simulink model "CrCtl_StM"  (R2016b)
settings: configuration reference "CodeGenConfigSet" (kept outside this file)
values from neighbouring files (symbols this model uses):
  CrCtl_aAccThres_C = Calibration.Parameter    [init_CrCtl_StM.m]
  CrCtl_aDeclThres_C = Calibration.Parameter    [init_CrCtl_StM.m]
  CrCtl_facRmpSlpAcc_C = Calibration.Parameter    [init_CrCtl_StM.m]
  CrCtl_facRmpSlpDecl_C = Calibration.Parameter    [init_CrCtl_StM.m]
  CrCtl_facRmpSlpRes_C = Calibration.Parameter    [init_CrCtl_StM.m]
  CrCtl_swtOffTipDwnTrqLim_C = Calibration.Parameter    [init_CrCtl_StM.m]
  CrCtl_swtOffTipUpTrqLim_C = Calibration.Parameter    [init_CrCtl_StM.m]
  CrCtl_trqLimOffsetAcc_C = Calibration.Parameter    [init_CrCtl_StM.m]
  CrCtl_trqLimOffsetDecl_C = Calibration.Parameter    [init_CrCtl_StM.m]
  CrCtl_vDvtMaxAccDecl_C = Calibration.Parameter    [init_CrCtl_StM.m]
  CrCtl_vMaxDvtAcc_C = Calibration.Parameter    [init_CrCtl_StM.m]
  CrCtl_vMaxDvtDecl_C = Calibration.Parameter    [init_CrCtl_StM.m]
  CrCtl_vMaxDvtResAbv_C = Calibration.Parameter    [init_CrCtl_StM.m]
  CrCtl_vMaxDvtResBlw_C = Calibration.Parameter    [init_CrCtl_StM.m]
  CrCtl_vTipDwnDvtn_C = Calibration.Parameter    [init_CrCtl_StM.m]
  CrCtl_vTipDwnLoLim_C = Calibration.Parameter    [init_CrCtl_StM.m]
  CrCtl_vTipDwnUpLim_C = Calibration.Parameter    [init_CrCtl_StM.m]
  CrCtl_vTipStp_C = Calibration.Parameter    [init_CrCtl_StM.m]
  CrCtl_vTipUpDvtn_C = Calibration.Parameter    [init_CrCtl_StM.m]
  CrCtl_vTipUpLoLim_C = Calibration.Parameter    [init_CrCtl_StM.m]
  CrCtl_vTipUpUpLim_C = Calibration.Parameter    [init_CrCtl_StM.m]
  MoFDrAs_vCCtlMinCalMsg_C = Calibration.Parameter    [init_CrCtl_StM.m]
  VEL_ZERO = fi(0,VehSpeed_km_h)    [init_CrCtl_StM.m]
undefined symbols (not defined in the file or in its folder): CrCtl_stLck_conv, CrCtl_StM_DT, CrCtl_stShOff_conv, CrCtl_stSub_conv, CruiseCtl_State_conv
libraries: CXLib x15
(part 2 of 2)

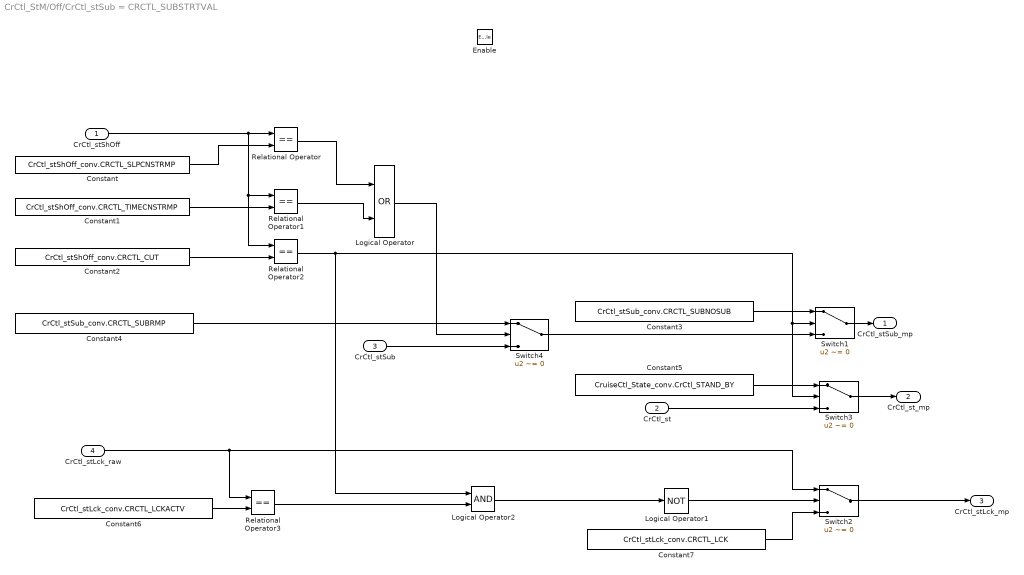
== system CrCtl_StM/Off/CrCtl_stSub = CRCTL_SUBSTRTVAL ==
  "CrCtl_stShOff " : Inport
  CrCtl_st : Inport  Port=2
  CrCtl_stSub : Inport  Port=3
  CrCtl_stLck_raw : Inport  Port=4
  Enable : EnablePort
  Constant : Constant  Value=CrCtl_stShOff_conv.CRCTL_SLPCNSTRMP
  Constant1 : Constant  Value=CrCtl_stShOff_conv.CRCTL_TIMECNSTRMP
  Constant2 : Constant  Value=CrCtl_stShOff_conv.CRCTL_CUT
  Constant3 : Constant  Value=CrCtl_stSub_conv.CRCTL_SUBNOSUB
  Constant4 : Constant  Value=CrCtl_stSub_conv.CRCTL_SUBRMP
  Constant5 : Constant  Value=CruiseCtl_State_conv.CrCtl_STAND_BY
  Constant6 : Constant  Value=CrCtl_stLck_conv.CRCTL_LCKACTV
  Constant7 : Constant  Value=CrCtl_stLck_conv.CRCTL_LCK
  Logical Operator : Logic  Operator=OR  AllPortsSameDT=off  OutDataTypeStr=boolean
  Logical Operator1 : Logic  Operator=NOT  AllPortsSameDT=off  OutDataTypeStr=boolean
  Logical Operator2 : Logic  AllPortsSameDT=off  OutDataTypeStr=boolean
  Relational Operator{,1..3} (4 alike) : RelationalOperator  Operator===  OutDataTypeStr=boolean  RndMeth=Simplest
  Switch{1..4} (4 alike) : Switch  Criteria=u2 ~= 0
  CrCtl_stSub_mp : Outport
  CrCtl_st_mp : Outport  Port=2
  CrCtl_stLck_mp : Outport  Port=3
  wires:
  Relational Operator1/1 -> Logical Operator/2
  Constant4/1 -> Switch4/1
  Switch4/1 -> Switch1/3
  Relational Operator2/1 -> Switch1/2, Switch3/2, Logical Operator2/1
  Constant3/1 -> Switch1/1
  Switch3/1 -> CrCtl_st_mp/1
  Constant7/1 -> Switch2/3
  Logical Operator/1 -> Switch4/2
  Constant5/1 -> Switch3/1
  Switch1/1 -> CrCtl_stSub_mp/1
  CrCtl_stLck_raw/1 -> Relational Operator3/1, Switch2/1
  Relational Operator/1 -> Logical Operator/1
  Constant2/1 -> Relational Operator2/2
  "CrCtl_stShOff "/1 -> Relational Operator1/1, Relational Operator2/1, Relational Operator/1
  Logical Operator2/1 -> Logical Operator1/1
  Constant6/1 -> Relational Operator3/2
  Logical Operator1/1 -> Switch2/2
  Constant1/1 -> Relational Operator1/2
  Constant/1 -> Relational Operator/2
  Relational Operator3/1 -> Logical Operator2/2
  Switch2/1 -> CrCtl_stLck_mp/1
  CrCtl_stSub/1 -> Switch4/3
  CrCtl_st/1 -> Switch3/3

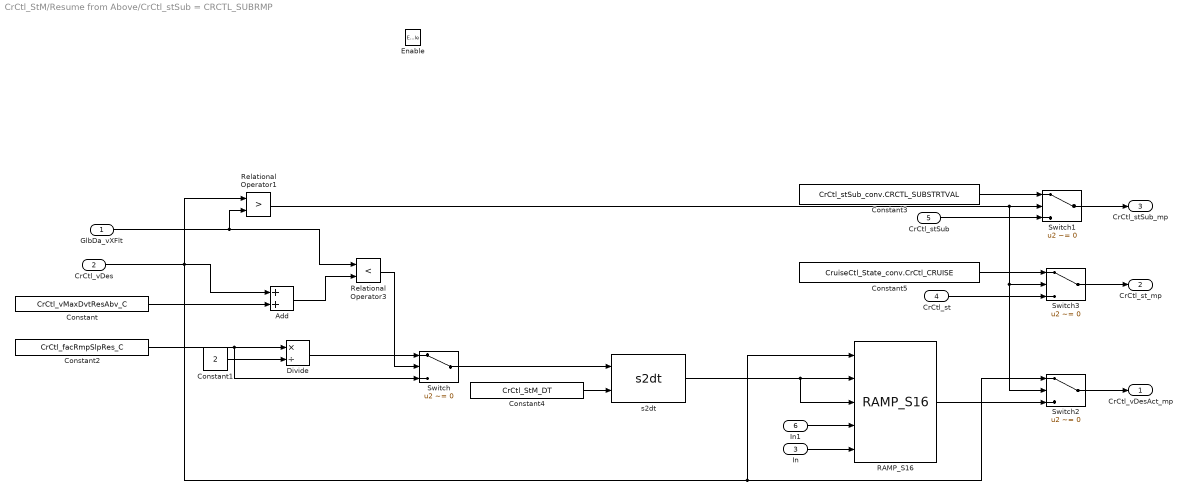
== system CrCtl_StM/Resume from Above/CrCtl_stSub = CRCTL_SUBRMP ==
  GlbDa_vXFlt : Inport
  CrCtl_vDes : Inport  Port=2
  In : Inport  Port=3
  CrCtl_st : Inport  Port=4
  CrCtl_stSub : Inport  Port=5
  In1 : Inport  Port=6
  Enable : EnablePort
  Add : Sum
  Constant : Constant  Value=CrCtl_vMaxDvtResAbv_C
  Constant1 : Constant  Value=2  OutDataTypeStr=Inherit: Inherit via back propagation
  Constant2 : Constant  Value=CrCtl_facRmpSlpRes_C
  Constant3 : Constant  Value=CrCtl_stSub_conv.CRCTL_SUBSTRTVAL
  Constant4 : Constant  Value=CrCtl_StM_DT
  Constant5 : Constant  Value=CruiseCtl_State_conv.CrCtl_CRUISE
  Divide : Product  Inputs=*/  OutDataTypeStr=Acc_m_s2
  RAMP_S16 : CXLib/RAMP_S16
  Relational Operator1 : RelationalOperator  Operator=>  OutDataTypeStr=boolean  RndMeth=Simplest
  Relational Operator3 : RelationalOperator  Operator=<  OutDataTypeStr=boolean  RndMeth=Simplest
  Switch{,1..3} (4 alike) : Switch  Criteria=u2 ~= 0
  s2dt : CXLib/s2dt
  CrCtl_vDesAct_mp : Outport
  CrCtl_st_mp : Outport  Port=2
  CrCtl_stSub_mp : Outport  Port=3
  wires:
  GlbDa_vXFlt/1 -> Relational Operator1/2, Relational Operator3/1
  Constant/1 -> Add/2
  Add/1 -> Relational Operator3/2
  Constant1/1 -> Divide/2
  Constant2/1 -> Switch/3, Divide/1
  Relational Operator3/1 -> Switch/2
  Divide/1 -> Switch/1
  s2dt/1 -> RAMP_S16/3, RAMP_S16/2
  Switch/1 -> s2dt/1
  Constant4/1 -> s2dt/2
  RAMP_S16/1 -> Switch2/3
  Constant3/1 -> Switch1/1
  Switch1/1 -> CrCtl_stSub_mp/1
  Switch3/1 -> CrCtl_st_mp/1
  Constant5/1 -> Switch3/1
  Switch2/1 -> CrCtl_vDesAct_mp/1
  Relational Operator1/1 -> Switch2/2, Switch3/2, Switch1/2
  CrCtl_vDes/1 -> RAMP_S16/1, Switch2/1, Relational Operator1/1, Add/1
  CrCtl_st/1 -> Switch3/3
  CrCtl_stSub/1 -> Switch1/3
  In/1 -> RAMP_S16/5
  In1/1 -> RAMP_S16/4

== system CrCtl_StM/Resume from Above/CrCtl_stSub = CRCTL_SUBSTRTVAL ==
  GlbDa_vXFlt : Inport
  CrCtl_vDes : Inport  Port=2
  CrCtl_vMax : Inport  Port=3
  Enable : EnablePort
  Constant3 : Constant  Value=CrCtl_stSub_conv.CRCTL_SUBRMP
  MinMax : MinMax  Function=max  Inputs=2
  MinMax1 : MinMax  Inputs=2
  CrCtl_stSub_mp : Outport
  CrCtl_vDesAct : Outport  Port=2
  wires:
  Constant3/1 -> CrCtl_stSub_mp/1
  GlbDa_vXFlt/1 -> MinMax/1
  CrCtl_vDes/1 -> MinMax/2
  MinMax/1 -> MinMax1/1
  MinMax1/1 -> CrCtl_vDesAct/1
  CrCtl_vMax/1 -> MinMax1/2

== system CrCtl_StM/Resume from Below/CrCtl_stSub = CRCTL_SUBPRECRUISE ==
  GlbDa_vXFlt : Inport
  CrCtl_vDes : Inport  Port=2
  CrCtl_stSuspRamp : Inport  Port=3
  CrCtl_stSub : Inport  Port=4
  CrCtl_st : Inport  Port=5
  Enable : EnablePort
  Constant : Constant  Value=0  OutDataTypeStr=uint8
  Constant1 : Constant  Value=CruiseCtl_State_conv.CrCtl_CRUISE
  Constant3 : Constant  Value=CrCtl_stSub_conv.CRCTL_SUBSTRTVAL
  Data Type Conversion : DataTypeConversion  OutDataTypeStr=uint8
  Logical Operator1 : Logic  AllPortsSameDT=off  OutDataTypeStr=boolean
  Relational Operator1 : RelationalOperator  Operator===  OutDataTypeStr=boolean  RndMeth=Simplest
  Relational Operator2 : RelationalOperator  OutDataTypeStr=boolean  RndMeth=Simplest
  Switch1 : Switch  Criteria=u2 ~= 0
  Switch3 : Switch  Criteria=u2 ~= 0
  CrCtl_vDesAct_mp : Outport
  CrCtl_st_mp : Outport  Port=2
  CrCtl_stSub_mp : Outport  Port=3
  wires:
  Switch1/1 -> CrCtl_stSub_mp/1
  Constant3/1 -> Switch1/1
  Logical Operator1/1 -> Switch3/2, Switch1/2
  Relational Operator2/1 -> Logical Operator1/2
  Relational Operator1/1 -> Logical Operator1/1
  CrCtl_vDes/1 -> CrCtl_vDesAct_mp/1, Relational Operator2/2
  GlbDa_vXFlt/1 -> Relational Operator2/1
  CrCtl_stSuspRamp/1 -> Data Type Conversion/1
  Constant/1 -> Relational Operator1/2
  Switch3/1 -> CrCtl_st_mp/1
  Constant1/1 -> Switch3/1
  CrCtl_stSub/1 -> Switch1/3
  CrCtl_st/1 -> Switch3/3
  Data Type Conversion/1 -> Relational Operator1/1

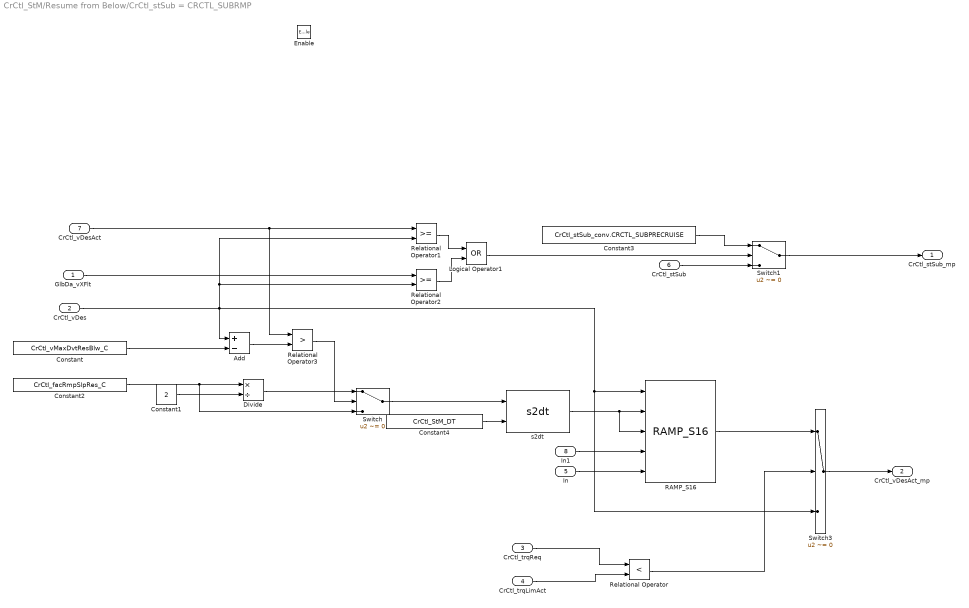
== system CrCtl_StM/Resume from Below/CrCtl_stSub = CRCTL_SUBRMP ==
  GlbDa_vXFlt : Inport
  CrCtl_vDes : Inport  Port=2
  CrCtl_trqReq : Inport  Port=3
  CrCtl_trqLimAct : Inport  Port=4
  In : Inport  Port=5
  CrCtl_stSub : Inport  Port=6
  CrCtl_vDesAct : Inport  Port=7
  In1 : Inport  Port=8
  Enable : EnablePort
  Add : Sum  Inputs=+-
  Constant : Constant  Value=CrCtl_vMaxDvtResBlw_C
  Constant1 : Constant  Value=2  OutDataTypeStr=Inherit: Inherit via back propagation
  Constant2 : Constant  Value=CrCtl_facRmpSlpRes_C
  Constant3 : Constant  Value=CrCtl_stSub_conv.CRCTL_SUBPRECRUISE
  Constant4 : Constant  Value=CrCtl_StM_DT
  Divide : Product  Inputs=*/  OutDataTypeStr=Acc_m_s2
  Logical Operator1 : Logic  Operator=OR  AllPortsSameDT=off  OutDataTypeStr=boolean
  RAMP_S16 : CXLib/RAMP_S16
  Relational Operator : RelationalOperator  Operator=<  OutDataTypeStr=boolean  RndMeth=Simplest
  Relational Operator1 : RelationalOperator  OutDataTypeStr=boolean  RndMeth=Simplest
  Relational Operator2 : RelationalOperator  OutDataTypeStr=boolean  RndMeth=Simplest
  Relational Operator3 : RelationalOperator  Operator=>  OutDataTypeStr=boolean  RndMeth=Simplest
  Switch : Switch  Criteria=u2 ~= 0
  Switch1 : Switch  Criteria=u2 ~= 0
  Switch3 : Switch  Criteria=u2 ~= 0
  s2dt : CXLib/s2dt
  CrCtl_stSub_mp : Outport
  CrCtl_vDesAct_mp : Outport  Port=2
  wires:
  GlbDa_vXFlt/1 -> Relational Operator2/1
  CrCtl_trqReq/1 -> Relational Operator/1
  CrCtl_trqLimAct/1 -> Relational Operator/2
  Constant/1 -> Add/2
  Add/1 -> Relational Operator3/2
  Constant1/1 -> Divide/2
  Constant2/1 -> Switch/3, Divide/1
  Relational Operator3/1 -> Switch/2
  Divide/1 -> Switch/1
  s2dt/1 -> RAMP_S16/3, RAMP_S16/2
  Switch/1 -> s2dt/1
  Constant4/1 -> s2dt/2
  Relational Operator/1 -> Switch3/2
  CrCtl_vDesAct/1 -> Relational Operator3/1, Relational Operator1/1
  Relational Operator1/1 -> Logical Operator1/1
  Relational Operator2/1 -> Logical Operator1/2
  Logical Operator1/1 -> Switch1/2
  Constant3/1 -> Switch1/1
  Switch1/1 -> CrCtl_stSub_mp/1
  CrCtl_stSub/1 -> Switch1/3
  In/1 -> RAMP_S16/5
  CrCtl_vDes/1 -> Switch3/3, RAMP_S16/1, Relational Operator2/2, Relational Operator1/2, Add/1
  RAMP_S16/1 -> Switch3/1
  Switch3/1 -> CrCtl_vDesAct_mp/1
  In1/1 -> RAMP_S16/4

== system CrCtl_StM/Resume from Below/CrCtl_stSub = CRCTL_SUBSTRTVAL ==
  GlbDa_vXFlt : Inport
  CrCtl_vDes : Inport  Port=2
  Enable : EnablePort
  Constant3 : Constant  Value=CrCtl_stSub_conv.CRCTL_SUBSTRTVAL
  MinMax : MinMax  Inputs=2
  CrCtl_stSub_mp : Outport
  CrCtl_vDesAct : Outport  Port=2
  wires:
  Constant3/1 -> CrCtl_stSub_mp/1
  GlbDa_vXFlt/1 -> MinMax/1
  CrCtl_vDes/1 -> MinMax/2
  MinMax/1 -> CrCtl_vDesAct/1

== system CrCtl_StM/Stand by/CRCTL_SUBNOSUB ==
  Enable : EnablePort

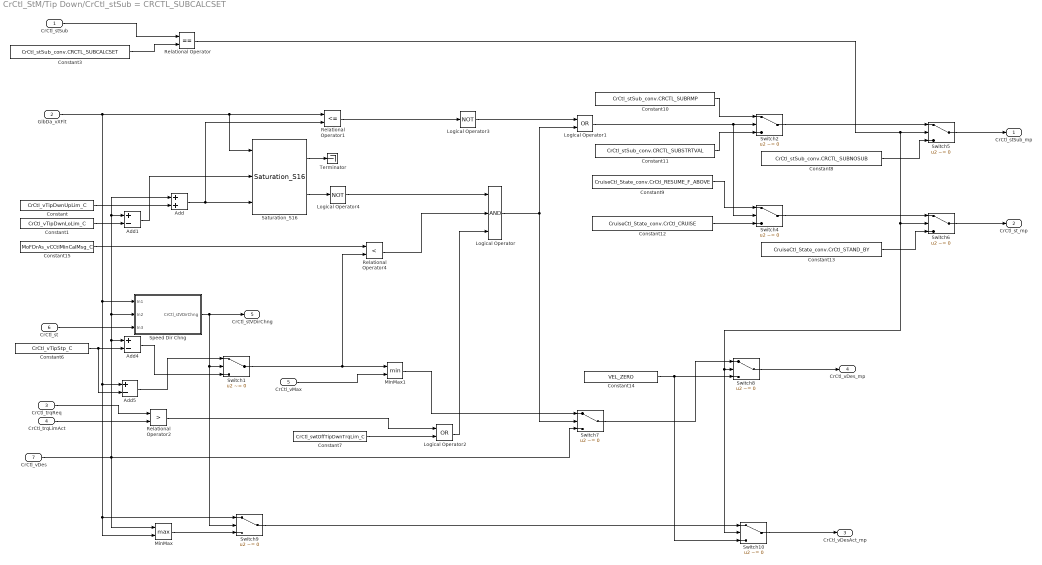
== system CrCtl_StM/Tip Down/CrCtl_stSub = CRCTL_SUBCALCSET ==
  CrCtl_stSub : Inport
  GlbDa_vXFlt : Inport  Port=2
  CrCtl_trqReq : Inport  Port=3
  CrCtl_trqLimAct : Inport  Port=4
  CrCtl_vMax : Inport  Port=5
  CrCtl_st : Inport  Port=6
  CrCtl_vDes : Inport  Port=7
  Add : Sum
  Add1 : Sum  Inputs=+-
  Add4 : Sum  Inputs=+-
  Add5 : Sum  Inputs=+-
  Constant : Constant  Value=CrCtl_vTipDwnUpLim_C
  Constant1 : Constant  Value=CrCtl_vTipDwnLoLim_C
  Constant10 : Constant  Value=CrCtl_stSub_conv.CRCTL_SUBRMP
  Constant11 : Constant  Value=CrCtl_stSub_conv.CRCTL_SUBSTRTVAL
  Constant12 : Constant  Value=CruiseCtl_State_conv.CrCtl_CRUISE
  Constant13 : Constant  Value=CruiseCtl_State_conv.CrCtl_STAND_BY
  Constant14 : Constant  Value=VEL_ZERO  OutDataTypeStr=VehSpeed_km_h
  Constant15 : Constant  Value=MoFDrAs_vCCtlMinCalMsg_C
  Constant3 : Constant  Value=CrCtl_stSub_conv.CRCTL_SUBCALCSET
  Constant6 : Constant  Value=CrCtl_vTipStp_C
  Constant7 : Constant  Value=CrCtl_swtOffTipDwnTrqLim_C
  Constant8 : Constant  Value=CrCtl_stSub_conv.CRCTL_SUBNOSUB
  Constant9 : Constant  Value=CruiseCtl_State_conv.CrCtl_RESUME_F_ABOVE
  Logical Operator : Logic  Inputs=3  AllPortsSameDT=off  OutDataTypeStr=boolean
  Logical Operator1 : Logic  Operator=OR  AllPortsSameDT=off  OutDataTypeStr=boolean
  Logical Operator2 : Logic  Operator=OR  AllPortsSameDT=off  OutDataTypeStr=boolean
  Logical Operator3 : Logic  Operator=NOT  AllPortsSameDT=off  OutDataTypeStr=boolean
  Logical Operator4 : Logic  Operator=NOT  AllPortsSameDT=off  OutDataTypeStr=boolean
  MinMax : MinMax  Function=max  Inputs=2
  MinMax1 : MinMax  Inputs=2
  Relational Operator : RelationalOperator  Operator===  OutDataTypeStr=boolean  RndMeth=Simplest
  Relational Operator1 : RelationalOperator  Operator=<=  OutDataTypeStr=boolean  RndMeth=Simplest
  Relational Operator2 : RelationalOperator  Operator=>  OutDataTypeStr=boolean  RndMeth=Simplest
  Relational Operator4 : RelationalOperator  Operator=<  OutDataTypeStr=boolean  RndMeth=Simplest
  Saturation_S16 : CXLib/Saturation_S16
  Speed Dir Chng : Subsystem
  Switch{1..2,4..10} (9 alike) : Switch  Criteria=u2 ~= 0
  Terminator : Terminator
  CrCtl_stSub_mp : Outport
  CrCtl_st_mp : Outport  Port=2
  CrCtl_vDesAct_mp : Outport  Port=3
  CrCtl_vDes_mp : Outport  Port=4
  CrCtl_stVDirChng : Outport  Port=5
  wires:
  Constant7/1 -> Logical Operator2/2
  Logical Operator2/1 -> Logical Operator/3
  Add5/1 -> Switch1/1
  Relational Operator1/1 -> Logical Operator3/1
  Add/1 -> Saturation_S16/3, Relational Operator1/2
  Constant1/1 -> Add1/2
  Constant/1 -> Add/2
  Constant6/1 -> Add5/2, Add4/2
  CrCtl_stSub/1 -> Relational Operator/1
  Add4/1 -> Switch1/3
  Switch1/1 -> Relational Operator4/2, MinMax1/1
  CrCtl_vMax/1 -> MinMax1/2
  Constant3/1 -> Relational Operator/2
  Logical Operator/1 -> Switch7/2, Logical Operator1/2
  CrCtl_trqReq/1 -> Relational Operator2/1
  CrCtl_trqLimAct/1 -> Relational Operator2/2
  Relational Operator2/1 -> Logical Operator2/1
  Constant15/1 -> Relational Operator4/1
  Switch4/1 -> Switch6/1
  Relational Operator4/1 -> Logical Operator/2
  MinMax1/1 -> Switch7/1
  Switch6/1 -> CrCtl_st_mp/1
  Switch7/1 -> Switch8/1
  Switch10/1 -> CrCtl_vDesAct_mp/1
  Constant14/1 -> Switch10/3, Switch8/3
  CrCtl_vDes/1 -> Switch7/3, Add1/1, Add/1, Speed Dir Chng/2(In2), Add4/1, MinMax/1
  Switch9/1 -> Switch10/1
  Logical Operator1/1 -> Switch4/2, Switch2/2
  Switch2/1 -> Switch5/1
  Constant11/1 -> Switch2/3
  CrCtl_st/1 -> Speed Dir Chng/3(In3)
  Relational Operator/1 -> Switch8/2, Switch10/2, Switch6/2, Switch5/2
  Logical Operator3/1 -> Logical Operator1/1
  Switch8/1 -> CrCtl_vDes_mp/1
  Constant8/1 -> Switch5/3
  Constant10/1 -> Switch2/1
  Constant12/1 -> Switch4/3
  MinMax/1 -> Switch9/3
  Constant9/1 -> Switch4/1
  Constant13/1 -> Switch6/3
  Speed Dir Chng/1(CrCtl_stVDirChng) -> CrCtl_stVDirChng/1, Switch9/2, Switch1/2
  Switch5/1 -> CrCtl_stSub_mp/1
  GlbDa_vXFlt/1 -> Speed Dir Chng/1(In1), Add5/1, Switch9/1, MinMax/2, Saturation_S16/1, Relational Operator1/1
  Add1/1 -> Saturation_S16/2
  Saturation_S16/2 -> Logical Operator4/1
  Logical Operator4/1 -> Logical Operator/1
  Saturation_S16/1 -> Terminator/1

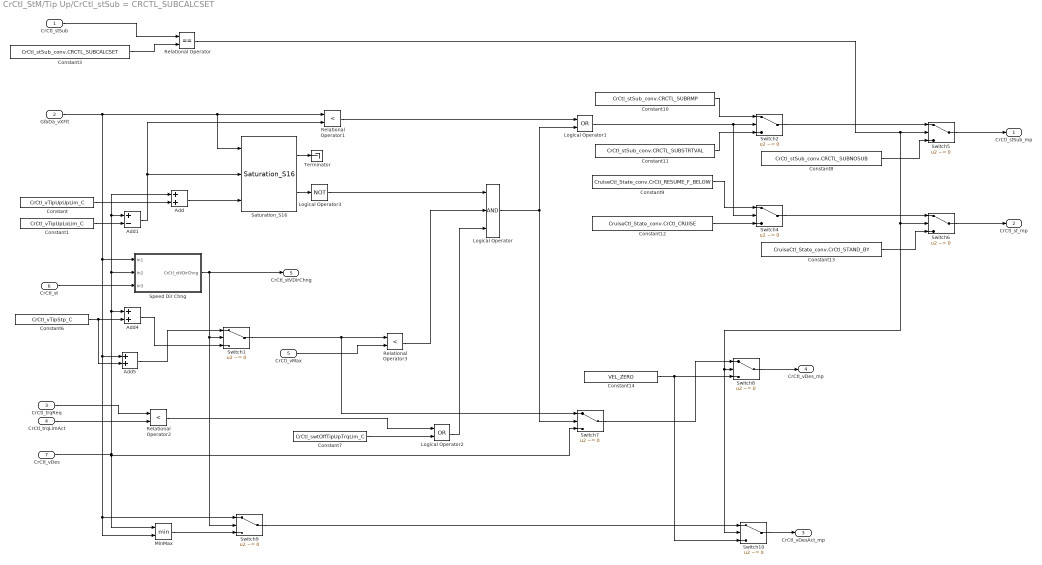
== system CrCtl_StM/Tip Up/CrCtl_stSub = CRCTL_SUBCALCSET ==
  CrCtl_stSub : Inport
  GlbDa_vXFlt : Inport  Port=2
  CrCtl_trqReq : Inport  Port=3
  CrCtl_trqLimAct : Inport  Port=4
  CrCtl_vMax : Inport  Port=5
  CrCtl_st : Inport  Port=6
  CrCtl_vDes : Inport  Port=7
  Add : Sum
  Add1 : Sum  Inputs=+-
  Add4 : Sum
  Add5 : Sum
  Constant : Constant  Value=CrCtl_vTipUpUpLim_C
  Constant1 : Constant  Value=CrCtl_vTipUpLoLim_C
  Constant10 : Constant  Value=CrCtl_stSub_conv.CRCTL_SUBRMP
  Constant11 : Constant  Value=CrCtl_stSub_conv.CRCTL_SUBSTRTVAL
  Constant12 : Constant  Value=CruiseCtl_State_conv.CrCtl_CRUISE
  Constant13 : Constant  Value=CruiseCtl_State_conv.CrCtl_STAND_BY
  Constant14 : Constant  Value=VEL_ZERO  OutDataTypeStr=VehSpeed_km_h
  Constant3 : Constant  Value=CrCtl_stSub_conv.CRCTL_SUBCALCSET
  Constant6 : Constant  Value=CrCtl_vTipStp_C
  Constant7 : Constant  Value=CrCtl_swtOffTipUpTrqLim_C
  Constant8 : Constant  Value=CrCtl_stSub_conv.CRCTL_SUBNOSUB
  Constant9 : Constant  Value=CruiseCtl_State_conv.CrCtl_RESUME_F_BELOW
  Logical Operator : Logic  Inputs=3  AllPortsSameDT=off  OutDataTypeStr=boolean
  Logical Operator1 : Logic  Operator=OR  AllPortsSameDT=off  OutDataTypeStr=boolean
  Logical Operator2 : Logic  Operator=OR  AllPortsSameDT=off  OutDataTypeStr=boolean
  Logical Operator3 : Logic  Operator=NOT  AllPortsSameDT=off  OutDataTypeStr=boolean
  MinMax : MinMax  Inputs=2
  Relational Operator : RelationalOperator  Operator===  OutDataTypeStr=boolean  RndMeth=Simplest
  Relational Operator1 : RelationalOperator  Operator=<  OutDataTypeStr=boolean  RndMeth=Simplest
  Relational Operator2 : RelationalOperator  Operator=<  OutDataTypeStr=boolean  RndMeth=Simplest
  Relational Operator3 : RelationalOperator  Operator=<  OutDataTypeStr=boolean  RndMeth=Simplest
  Saturation_S16 : CXLib/Saturation_S16
  Speed Dir Chng : Subsystem
  Switch{1..2,4..10} (9 alike) : Switch  Criteria=u2 ~= 0
  Terminator : Terminator
  CrCtl_stSub_mp : Outport
  CrCtl_st_mp : Outport  Port=2
  CrCtl_vDesAct_mp : Outport  Port=3
  CrCtl_vDes_mp : Outport  Port=4
  CrCtl_stVDirChng : Outport  Port=5
  wires:
  Constant6/1 -> Add5/2, Add4/2
  CrCtl_stSub/1 -> Relational Operator/1
  GlbDa_vXFlt/1 -> Speed Dir Chng/1(In1), Add5/1, Switch9/1, MinMax/2, Saturation_S16/1, Relational Operator1/1
  Constant3/1 -> Relational Operator/2
  Logical Operator/1 -> Switch7/2, Logical Operator1/2
  Constant/1 -> Add/2
  Constant1/1 -> Add1/2
  Switch10/1 -> CrCtl_vDesAct_mp/1
  Constant10/1 -> Switch2/1
  Relational Operator3/1 -> Logical Operator/2
  CrCtl_trqReq/1 -> Relational Operator2/1
  CrCtl_trqLimAct/1 -> Relational Operator2/2
  Logical Operator2/1 -> Logical Operator/3
  Relational Operator1/1 -> Logical Operator1/1
  Constant8/1 -> Switch5/3
  Add5/1 -> Switch1/1
  Switch2/1 -> Switch5/1
  Switch4/1 -> Switch6/1
  Constant14/1 -> Switch10/3, Switch8/3
  Switch7/1 -> Switch8/1
  CrCtl_vDes/1 -> Switch7/3, MinMax/1, Speed Dir Chng/2(In2), Add1/1, Add/1, Add4/1
  Relational Operator/1 -> Switch8/2, Switch10/2, Switch6/2, Switch5/2
  Logical Operator1/1 -> Switch4/2, Switch2/2
  Constant12/1 -> Switch4/3
  Switch5/1 -> CrCtl_stSub_mp/1
  Constant9/1 -> Switch4/1
  Add4/1 -> Switch1/3
  MinMax/1 -> Switch9/3
  Relational Operator2/1 -> Logical Operator2/1
  Switch1/1 -> Switch7/1, Relational Operator3/1
  Constant11/1 -> Switch2/3
  Constant7/1 -> Logical Operator2/2
  Switch9/1 -> Switch10/1
  CrCtl_vMax/1 -> Relational Operator3/2
  Constant13/1 -> Switch6/3
  Switch6/1 -> CrCtl_st_mp/1
  Switch8/1 -> CrCtl_vDes_mp/1
  CrCtl_st/1 -> Speed Dir Chng/3(In3)
  Speed Dir Chng/1(CrCtl_stVDirChng) -> CrCtl_stVDirChng/1, Switch9/2, Switch1/2
  Add1/1 -> Saturation_S16/2, Relational Operator1/2
  Add/1 -> Saturation_S16/3
  Saturation_S16/1 -> Terminator/1
  Saturation_S16/2 -> Logical Operator3/1
  Logical Operator3/1 -> Logical Operator/1

== system CrCtl_StM/Tip Down/CrCtl_stSub = CRCTL_SUBCALCSET/Speed Dir Chng ==
  In1 : Inport
  In2 : Inport  Port=2
  In3 : Inport  Port=3
  Add5 : Sum  Inputs=+-
  Constant1 : Constant  Value=CruiseCtl_State_conv.CrCtl_ACCELERATION
  Constant13 : Constant  Value=CruiseCtl_State_conv.CrCtl_RESUME_F_BELOW
  Constant2 : Constant  Value=CruiseCtl_State_conv.CrCtl_TIP_UP
  Constant3 : Constant  Value=CrCtl_vTipDwnDvtn_C
  Logical Operator : Logic  Operator=OR  Inputs=3  AllPortsSameDT=off  OutDataTypeStr=boolean
  Logical Operator2 : Logic  AllPortsSameDT=off  OutDataTypeStr=boolean
  Relational Operator1 : RelationalOperator  Operator===  OutDataTypeStr=boolean  RndMeth=Simplest
  Relational Operator2 : RelationalOperator  Operator===  OutDataTypeStr=boolean  RndMeth=Simplest
  Relational Operator3 : RelationalOperator  Operator===  OutDataTypeStr=boolean  RndMeth=Simplest
  Relational Operator4 : RelationalOperator  Operator=>  OutDataTypeStr=boolean  RndMeth=Simplest
  CrCtl_stVDirChng : Outport
  wires:
  In3/1 -> Relational Operator2/1, Relational Operator1/1, Relational Operator3/1
  Constant13/1 -> Relational Operator3/2
  Constant2/1 -> Relational Operator2/2
  Constant1/1 -> Relational Operator1/2
  Relational Operator3/1 -> Logical Operator/1
  Relational Operator1/1 -> Logical Operator/2
  Relational Operator2/1 -> Logical Operator/3
  Constant3/1 -> Add5/2
  In2/1 -> Add5/1
  In1/1 -> Relational Operator4/2
  Add5/1 -> Relational Operator4/1
  Logical Operator/1 -> Logical Operator2/1
  Relational Operator4/1 -> Logical Operator2/2
  Logical Operator2/1 -> CrCtl_stVDirChng/1

== system CrCtl_StM/Tip Up/CrCtl_stSub = CRCTL_SUBCALCSET/Speed Dir Chng ==
  In1 : Inport
  In2 : Inport  Port=2
  In3 : Inport  Port=3
  Add5 : Sum
  Constant1 : Constant  Value=CruiseCtl_State_conv.CrCtl_DECELERATION
  Constant13 : Constant  Value=CruiseCtl_State_conv.CrCtl_RESUME_F_ABOVE
  Constant2 : Constant  Value=CruiseCtl_State_conv.CrCtl_TIP_DOWN
  Constant3 : Constant  Value=CrCtl_vTipUpDvtn_C
  Logical Operator : Logic  Operator=OR  Inputs=3  AllPortsSameDT=off  OutDataTypeStr=boolean
  Logical Operator2 : Logic  AllPortsSameDT=off  OutDataTypeStr=boolean
  Relational Operator1 : RelationalOperator  Operator===  OutDataTypeStr=boolean  RndMeth=Simplest
  Relational Operator2 : RelationalOperator  Operator===  OutDataTypeStr=boolean  RndMeth=Simplest
  Relational Operator3 : RelationalOperator  Operator===  OutDataTypeStr=boolean  RndMeth=Simplest
  Relational Operator4 : RelationalOperator  Operator=<  OutDataTypeStr=boolean  RndMeth=Simplest
  CrCtl_stVDirChng : Outport
  wires:
  In3/1 -> Relational Operator2/1, Relational Operator1/1, Relational Operator3/1
  Constant13/1 -> Relational Operator3/2
  Constant2/1 -> Relational Operator2/2
  Constant1/1 -> Relational Operator1/2
  Relational Operator3/1 -> Logical Operator/1
  Relational Operator1/1 -> Logical Operator/2
  Relational Operator2/1 -> Logical Operator/3
  Constant3/1 -> Add5/2
  In2/1 -> Add5/1
  In1/1 -> Relational Operator4/2
  Add5/1 -> Relational Operator4/1
  Logical Operator/1 -> Logical Operator2/1
  Relational Operator4/1 -> Logical Operator2/2
  Logical Operator2/1 -> CrCtl_stVDirChng/1
